simulink model "DIshi1"  (R2020a)
settings: Solver=ode45  StartTime=0.0  StopTime=5E-4  RelTol=1e-6  AbsTol=1e-6
InitFcn:
  | R1 = 1000;
  | R2 = 20;
  | L = 25.3E-6;
  | C = 100E-9;
  | IS = 1E-8;
  | UT = 26E-3;
  | f = 0.15E+6;
settings Model: Creator=LKP  LastModifiedBy=peter
settings DataIOCC: OutputOption=SpecifiedOutputTimes  OutputTimes=0:1e-8:5e-4
settings DebuggingCC: AlgebraicLoopMsg=none  ArtificialAlgebraicLoopMsg=none

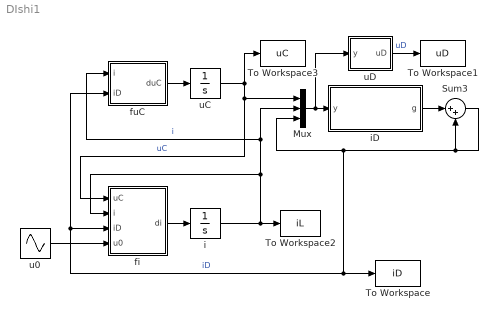
== system DIshi1 ==
  Mux : Mux  Inputs=3
  Sum3 : Sum  Inputs=|++
  To Workspace : ToWorkspace  VariableName=iD  SaveFormat=Timeseries  SampleTime=-1
  To Workspace1 : ToWorkspace  VariableName=uD  SaveFormat=Timeseries  SampleTime=-1
  To Workspace2 : ToWorkspace  VariableName=iL  SaveFormat=Timeseries  SampleTime=-1
  To Workspace3 : ToWorkspace  VariableName=uC  SaveFormat=Timeseries  SampleTime=-1
  fi : Subsystem
  fuC : Subsystem
  i : Integrator
  iD : Subsystem
      mask Display: disp('g(uC, i, iD)')
  u0 : Sin  Amplitude=-1  Frequency=2*pi*f  SampleTime=0
  uC : Integrator
  uD : Subsystem
  wires:
  i/1 -> fuC/1(i), Mux/2, fi/2(i), To Workspace2/1  "i"
  Sum3/1 -> Sum3/2, Mux/3, fuC/2(iD), fi/3(iD), To Workspace/1  "iD"
  uC/1 -> fi/1(uC), Mux/1, To Workspace3/1  "uC"
  iD/1(g) -> Sum3/1
  Mux/1 -> uD/1(y), iD/1(y)
  fuC/1(duC) -> uC/1
  fi/1(di) -> i/1
  uD/1(uD) -> To Workspace1/1  "uD"
  u0/1 -> fi/4(u0)

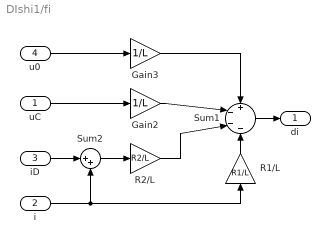
== system DIshi1/fi ==
  uC : Inport
  i : Inport  Port=2
  iD : Inport  Port=3
  u0 : Inport  Port=4
  Gain2 : Gain  Gain=1/L
  Gain3 : Gain  Gain=1/L
  R1/L : Gain  Gain=R1/L
  R2/L : Gain  Gain=R2/L
  Sum1 : Sum  Inputs=+---
  Sum2 : Sum  Inputs=|++
  di : Outport
  wires:
  Gain2/1 -> Sum1/2
  Sum1/1 -> di/1
  R1/L/1 -> Sum1/4
  i/1 -> R1/L/1, Sum2/2
  Sum2/1 -> R2/L/1
  uC/1 -> Gain2/1
  u0/1 -> Gain3/1
  R2/L/1 -> Sum1/3
  Gain3/1 -> Sum1/1
  iD/1 -> Sum2/1

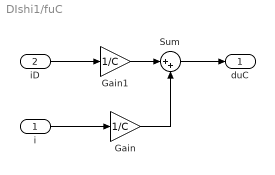
== system DIshi1/fuC ==
  i : Inport
  iD : Inport  Port=2
  Gain : Gain  Gain=1/C
  Gain1 : Gain  Gain=1/C
  Sum : Sum  Inputs=|++
  duC : Outport
  wires:
  i/1 -> Gain/1
  iD/1 -> Gain1/1
  Gain1/1 -> Sum/1
  Gain/1 -> Sum/2
  Sum/1 -> duC/1

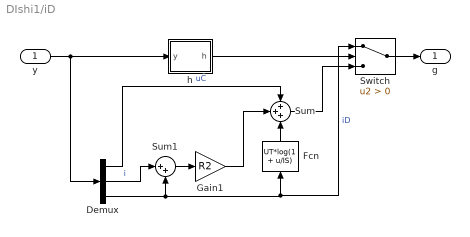
== system DIshi1/iD ==
  y : Inport
  Demux : Demux  Outputs=3
  Fcn : Fcn  Expr=UT*log(1 + u/IS)
  Gain1 : Gain  Gain=R2
  Sum : Sum  Inputs=+++
  Sum1 : Sum  Inputs=|++
  Switch : Switch  Criteria=u2 > Threshold
  h : Subsystem
  g : Outport
  wires:
  y/1 -> Demux/1, h/1(y)
  Switch/1 -> g/1
  h/1(h) -> Switch/2
  Demux/3 -> Switch/1, Fcn/1, Sum1/2  "iD"
  Demux/2 -> Sum1/1  "i"
  Sum1/1 -> Gain1/1
  Gain1/1 -> Sum/2
  Demux/1 -> Sum/1  "uC"
  Fcn/1 -> Sum/3
  Sum/1 -> Switch/3

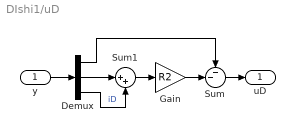
== system DIshi1/uD ==
  y : Inport
  Demux : Demux  Outputs=3
  Gain : Gain  Gain=R2
  Sum : Sum  Inputs=--|
  Sum1 : Sum  Inputs=|++
  uD : Outport
  wires:
  Demux/2 -> Sum1/1
  Sum/1 -> uD/1
  Demux/1 -> Sum/1
  Gain/1 -> Sum/2
  Sum1/1 -> Gain/1
  Demux/3 -> Sum1/2  "iD"
  y/1 -> Demux/1

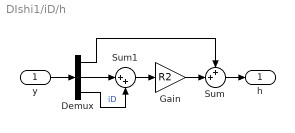
== system DIshi1/iD/h ==
  y : Inport
  Demux : Demux  Outputs=3
  Gain : Gain  Gain=R2
  Sum : Sum  Inputs=++|
  Sum1 : Sum  Inputs=|++
  h : Outport
  wires:
  Demux/2 -> Sum1/1
  Sum/1 -> h/1
  Demux/1 -> Sum/1
  Gain/1 -> Sum/2
  Sum1/1 -> Gain/1
  Demux/3 -> Sum1/2  "iD"
  y/1 -> Demux/1
